simulink model "test_variable_sl"  (R2020a)
settings: Solver=VariableStepAuto  StartTime=0.0  StopTime=1  RelTol=1e-3
settings Model: Creator=giova  LastModifiedBy=giova

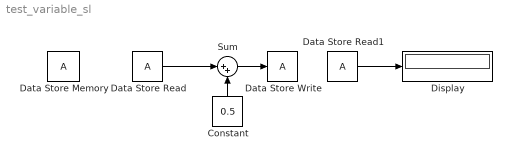
== system test_variable_sl ==
  Constant : Constant  Value=0.5
  Data Store Memory : DataStoreMemory  ReadBeforeWriteMsg=warning  WriteAfterWriteMsg=warning  WriteAfterReadMsg=warning  ShowAdditionalParam=off
  Data Store Read : DataStoreRead  SampleTime=-0
  Data Store Read1 : DataStoreRead
  Data Store Write : DataStoreWrite
  Display : Display
  Sum : Sum  Inputs=|++
  wires:
  Data Store Read/1 -> Sum/1
  Constant/1 -> Sum/2
  Sum/1 -> Data Store Write/1
  Data Store Read1/1 -> Display/1
